simulink model "power_13NodeTestFeeder_4VSC_PV_DEG_symmtrc_loads_"  (R2024b)
settings: Solver=ode15s  StartTime=0.0  StopTime=5  FixedStep=1e-6  MaxStep=1e-4  RelTol=1e-6  AbsTol=1e-8  EnableMultiTasking=on
PreLoadFcn:
  | %power_13NodeTestFeeder_init;
values from neighbouring files (symbols this model uses):
  a = 1.3    [init_para_with_symmtrc_loads.m]
  Cdc = 278e-3    (= 0.278)    [init_para_with_symmtrc_loads.m]
  fg = 60    [a01_scan_VSC_13_feeder.m]    (also in init_para_with_symmtrc_loads.m)
  Gn = 1000    [init_para_with_symmtrc_loads.m]
  H = 8    [init_para_with_symmtrc_loads.m]
  Ipv_n = Isc_n*(Rp+Rs)/Rp    (= 8.21426513558)    [init_para_with_symmtrc_loads.m]
  Isc_n = 8.21    [init_para_with_symmtrc_loads.m]
  k = 1.3806503e-23    [init_para_with_symmtrc_loads.m]    (also in ypm_plot_compare_ana_meas.m = 2)
  Kdroop = Sn/(Rdroop*60)    (= 4166666.66667)    [init_para_with_symmtrc_loads.m]
  KI = 0.0032    [init_para_with_symmtrc_loads.m]
  Ki_C = Rc/tau_C    (= 0.768)    [init_para_with_symmtrc_loads.m]
  Ki_DC = omega_DC^2*Cdc    [init_para_with_symmtrc_loads.m]
  ki_dvpp = kp_dvpp/Ti_dvpp    [init_para_with_symmtrc_loads.m]
  Ki_P = 1/(Ki_pq*tau_P)    [init_para_with_symmtrc_loads.m]
  Ki_PLL = Kp_PLL/tau_PLL    [init_para_with_symmtrc_loads.m]
  Kp_C = Lc/tau_C    (= 0.020372)    [init_para_with_symmtrc_loads.m]
  Kp_DC = 2*xi_DC*omega_DC*Cdc    [init_para_with_symmtrc_loads.m]
  kp_dvpp = -(2*Kdcgain)^-1    [init_para_with_symmtrc_loads.m]
  Kp_P = tau_C/(Ki_pq*tau_P)    [init_para_with_symmtrc_loads.m]
  Kp_PLL = xi_PLL*2*omega_PLL/Vp    [init_para_with_symmtrc_loads.m]
  KV = -0.123    [init_para_with_symmtrc_loads.m]
  kv_Vp = [ 1.021 1.042 1.0174]    [init_para_with_symmtrc_loads.m]
  KVmp = Vmp_n/Voc_n    (= 0.799392097264)    [init_para_with_symmtrc_loads.m]
  Lc = 20.372e-6    (= 2.0372e-05)    [init_para_with_symmtrc_loads.m]
  Lg = Xg /(2*pi*fg)    [init_para_with_symmtrc_loads.m]
  Np = 345    [init_para_with_symmtrc_loads.m]
  Ns = 45    [init_para_with_symmtrc_loads.m]
  Ns_cell = 54    [init_para_with_symmtrc_loads.m]
  p_jump_time = 5    [init_para_with_symmtrc_loads.m]
  p_jump_value = 2*-1e6    (= -2000000)    [init_para_with_symmtrc_loads.m]
  phi_vec = phi_vec_deg/180*pi    [init_para_with_symmtrc_loads.m]
  ppv_nom = 4.9687e+05    (= 496870)    [init_para_with_symmtrc_loads.m]
  q = 1.6021764e-19    [init_para_with_symmtrc_loads.m]
  Rc = 0.768e-3    (= 0.000768)    [init_para_with_symmtrc_loads.m]
  Rg = (U_rms^2 / S_sc) / (sqrt(1 + XoverR^2))    [init_para_with_symmtrc_loads.m]
  Rp = 425.405    [init_para_with_symmtrc_loads.m]
  Rs = 0.221    [init_para_with_symmtrc_loads.m]
  S_base_all = 1    [init_para_with_symmtrc_loads.m]
  Sn = 15e6    (= 15000000)    [init_para_with_symmtrc_loads.m]
  tau_PLL = 2*xi_PLL/omega_PLL    [init_para_with_symmtrc_loads.m]
  Tn = 25    [init_para_with_symmtrc_loads.m]
  Ts = T_ctrl/n_ctrl    [a01_scan_VSC_13_feeder.m]    (also in init_para_with_symmtrc_loads.m = 5e-05)
  U_rms = 4160    [init_para_with_symmtrc_loads.m]
  Vdc = 1200    [init_para_with_symmtrc_loads.m]
  Voc_n = 32.9    [init_para_with_symmtrc_loads.m]
  Vp = sqrt(2)*480/sqrt(3)    [a01_scan_VSC_13_feeder.m]    (also in init_para_with_symmtrc_loads.m = Ug*sqrt(2)/sqrt(3))
undefined symbols (not defined in the file or in its folder): j, Newton, para_grid, para_PVgeno, Raphson
libraries: spsabctoAlphaBetaZeroLib x141, spsPower3phInstantaneousLib x70, spsSeriesRLCBranchLib x44, spsThreePhaseVIMeasurementLib x27, slpidlib x24, spsThreePhaseSeriesRLCLoadLib x15, spsControlledVoltageSourceLib x15, spsMeanLib x9, spsCurrentMeasurementLib x8, spsControlledCurrentSourceLib x8, cstblocks x8, spsGroundLib x5
(part 2 of 10)

== system power_13NodeTestFeeder_4VSC_PV_DEG_symmtrc_loads_/PV1 dynamic Load2 ==
  delta_p : Inport
  Bus Selector : BusSelector  OutputSignals=Active power P (W)
  Constant : Constant  Value=ppv_nom
  Gain : Gain  Gain=[-1 0]
  PVG_at_634 : spsThreePhaseVIMeasurementLib/Three-Phase V-I Measurement  VoltageMeasurement=phase-to-ground  SetLabelV=off  LabelV=Vabc_634_pv  Vpu=off  VpuLL=off  CurrentMeasurement=yes  SetLabelI=off  LabelI=Iabc_634_pv  Ipu=off  Pbase=100e6  Vbase=4160  OutputType=Complex  PhasorSimulation=off  PSBequivalent=0
  Scope3 : Scope
  Sum : Sum  Inputs=|++
  Three-Phase Dynamic Load : spsThreePhaseDynamicLoadLib/Three-Phase Dynamic Load  NominalVoltage=[ para_grid.n634YgPQ.V_LN_rms(1)*sqrt(3) 60 ]  ActiveReactivePowers=[ppv_nom 0]  PositiveSequence=[1 0]  ExternalControl=on  NpNq=[1.3 2]  TimeConstants="[0  0  0  0]"  MinimumVoltage=0.7  Tfilter=1e-4  LoadFlowParameters=[4,0,0,0,0]
  a : PMIOPort  Side=Right
  b : PMIOPort  Port=2  Side=Right
  c : PMIOPort  Port=3  Side=Right
  tag scope: Iabc_675_pv=global, Vabc_675_pv=global
  wires:
  PVG_at_634/1 -> [Vabc_675_pv]
  Bus Selector/1 -> Scope3/1  "<Active power P (W)>"
  PVG_at_634/2 -> [Iabc_675_pv]
  Three-Phase Dynamic Load/1 -> Bus Selector/1
  Constant/1 -> Sum/2
  Gain/1 -> Three-Phase Dynamic Load/1
  Sum/1 -> Gain/1
  delta_p/1 -> Sum/1
  connections:
  PVG_at_634/LConn3 -- Three-Phase Dynamic Load/LConn3
  b/RConn1 -- PVG_at_634/RConn2
  a/RConn1 -- PVG_at_634/RConn1
  PVG_at_634/LConn2 -- Three-Phase Dynamic Load/LConn2
  c/RConn1 -- PVG_at_634/RConn3
  PVG_at_634/LConn1 -- Three-Phase Dynamic Load/LConn1

== system power_13NodeTestFeeder_4VSC_PV_DEG_symmtrc_loads_/PV1 dynamic Load3 ==
  delta_p : Inport
  Bus Selector : BusSelector  OutputSignals=Active power P (W)
  Constant : Constant  Value=ppv_nom
  Gain : Gain  Gain=[-1 0]
  PVG_at_634 : spsThreePhaseVIMeasurementLib/Three-Phase V-I Measurement  VoltageMeasurement=phase-to-ground  SetLabelV=off  LabelV=Vabc_634_pv  Vpu=off  VpuLL=off  CurrentMeasurement=yes  SetLabelI=off  LabelI=Iabc_634_pv  Ipu=off  Pbase=100e6  Vbase=4160  OutputType=Complex  PhasorSimulation=off  PSBequivalent=0
  Scope3 : Scope
  Sum : Sum  Inputs=|++
  Three-Phase Dynamic Load : spsThreePhaseDynamicLoadLib/Three-Phase Dynamic Load  NominalVoltage=[ para_grid.n634YgPQ.V_LN_rms(1)*sqrt(3) 60 ]  ActiveReactivePowers=[ppv_nom 0]  PositiveSequence=[1 0]  ExternalControl=on  NpNq=[1.3 2]  TimeConstants="[0  0  0  0]"  MinimumVoltage=0.7  Tfilter=1e-4  LoadFlowParameters=[4,0,0,0,0]
  a : PMIOPort  Side=Right
  b : PMIOPort  Port=2  Side=Right
  c : PMIOPort  Port=3  Side=Right
  tag scope: Iabc_680_pv=global, Vabc_680_pv=global
  wires:
  PVG_at_634/1 -> [Vabc_680_pv]
  Bus Selector/1 -> Scope3/1  "<Active power P (W)>"
  PVG_at_634/2 -> [Iabc_680_pv]
  Three-Phase Dynamic Load/1 -> Bus Selector/1
  Constant/1 -> Sum/2
  Gain/1 -> Three-Phase Dynamic Load/1
  Sum/1 -> Gain/1
  delta_p/1 -> Sum/1
  connections:
  PVG_at_634/LConn3 -- Three-Phase Dynamic Load/LConn3
  b/RConn1 -- PVG_at_634/RConn2
  a/RConn1 -- PVG_at_634/RConn1
  PVG_at_634/LConn2 -- Three-Phase Dynamic Load/LConn2
  c/RConn1 -- PVG_at_634/RConn3
  PVG_at_634/LConn1 -- Three-Phase Dynamic Load/LConn1

== system power_13NodeTestFeeder_4VSC_PV_DEG_symmtrc_loads_/PV2 dynamic Load ==
  delta_p : Inport
  Bus Selector : BusSelector  OutputSignals=Active power P (W)
  Constant : Constant  Value=ppv_nom
  Gain : Gain  Gain=[-1 0]
  PVG_at_634 : spsThreePhaseVIMeasurementLib/Three-Phase V-I Measurement  VoltageMeasurement=phase-to-ground  SetLabelV=off  LabelV=Vabc_634_pv  Vpu=off  VpuLL=off  CurrentMeasurement=yes  SetLabelI=off  LabelI=Iabc_634_pv  Ipu=off  Pbase=100e6  Vbase=4160  OutputType=Complex  PhasorSimulation=off  PSBequivalent=0
  Scope3 : Scope
  Sum : Sum  Inputs=|++
  Three-Phase Dynamic Load : spsThreePhaseDynamicLoadLib/Three-Phase Dynamic Load  NominalVoltage=[ para_grid.n634YgPQ.V_LN_rms(1)*sqrt(3) 60 ]  ActiveReactivePowers=[ppv_nom 0]  PositiveSequence=[1 0]  ExternalControl=on  NpNq=[1.3 2]  TimeConstants="[0  0  0  0]"  MinimumVoltage=0.7  Tfilter=1e-4  LoadFlowParameters=[4,0,0,0,0]
  a : PMIOPort  Side=Right
  b : PMIOPort  Port=2  Side=Right
  c : PMIOPort  Port=3  Side=Right
  tag scope: Iabc_672_pv=global, Vabc_672_pv=global
  wires:
  PVG_at_634/1 -> [Vabc_672_pv]
  Bus Selector/1 -> Scope3/1  "<Active power P (W)>"
  PVG_at_634/2 -> [Iabc_672_pv]
  Three-Phase Dynamic Load/1 -> Bus Selector/1
  Constant/1 -> Sum/2
  Gain/1 -> Three-Phase Dynamic Load/1
  delta_p/1 -> Sum/1
  Sum/1 -> Gain/1
  connections:
  PVG_at_634/LConn3 -- Three-Phase Dynamic Load/LConn3
  b/RConn1 -- PVG_at_634/RConn2
  a/RConn1 -- PVG_at_634/RConn1
  PVG_at_634/LConn2 -- Three-Phase Dynamic Load/LConn2
  c/RConn1 -- PVG_at_634/RConn3
  PVG_at_634/LConn1 -- Three-Phase Dynamic Load/LConn1

== system power_13NodeTestFeeder_4VSC_PV_DEG_symmtrc_loads_/PV_Geno_GFL_VSC_at_634 ==
  note: 5.23e5
  "PV-Geno with VSC_GFL_at_634     " : Subsystem
      settings: PortSchema="{\"entries\":[{\"content\":{\"sides\":[{\"content\":{\"connectorIds\":[\"LConn1\",\"LConn2\",\"LConn3\"]},\"type\":\"ConnectorPlacement.EquallySpacedRectSide\",\"uuid\":\"92a05cf9-a19b-475d-bffb-9406018f82f4\"},{\"content\":{\"connectorIds\":[\"In1\",\"In2\",\"In3\"],\"side\":\"RIGHT\"},\"type\":\"ConnectorPlacement.EquallySpacedRectSide\",\"uuid\":\"83076eb6-0a86-49d7-8932-035501cdc6f6\"},{\"content\":{\"side\":\"TOP\"},\"type\":\"ConnectorPlacement.EquallySpacedRectSide\",\"uuid\":\"ba2310df-ee07-4a5c-88ff-ef0f81658322\"}]},\"type\":\"ConnectorPlacement.EquallySpacedConnector\",\"uuid\":\"9e64c472-0dae-4bb4-8eb3-3329c328d412\"}],\"packageUris\":[\"http://schema.mathworks.com/mf0/Connector/R2020b\"],\"version\":\"1.0\"}"
  PVG_at_634 : spsThreePhaseVIMeasurementLib/Three-Phase V-I Measurement  VoltageMeasurement=phase-to-ground  SetLabelV=off  LabelV=Vabc_634_pv  Vpu=off  VpuLL=off  CurrentMeasurement=yes  SetLabelI=off  LabelI=Iabc_634_pv  Ipu=off  Pbase=100e6  Vbase=4160  OutputType=Complex  PhasorSimulation=off  PSBequivalent=0
  S Signalgenerator_at_1 : Subsystem
  a : PMIOPort  Side=Right
  b : PMIOPort  Port=2  Side=Right
  c : PMIOPort  Port=3  Side=Right
  tag scope: Iabc_634_pv=global, Vabc_634_pv=global
  wires:
  S Signalgenerator_at_1/1(S) -> "PV-Geno with VSC_GFL_at_634     "/3(S)
  PVG_at_634/2 -> [Iabc_634_pv], "PV-Geno with VSC_GFL_at_634     "/2(I_abc)
  PVG_at_634/1 -> [Vabc_634_pv], "PV-Geno with VSC_GFL_at_634     "/1(V_abc)
  connections:
  PVG_at_634/RConn2 -- b/RConn1
  "PV-Geno with VSC_GFL_at_634     "/LConn3 -- PVG_at_634/LConn3
  "PV-Geno with VSC_GFL_at_634     "/LConn1 -- PVG_at_634/LConn1
  "PV-Geno with VSC_GFL_at_634     "/LConn2 -- PVG_at_634/LConn2
  PVG_at_634/RConn1 -- a/RConn1
  PVG_at_634/RConn3 -- c/RConn1

== system power_13NodeTestFeeder_4VSC_PV_DEG_symmtrc_loads_/PV_Geno_GFL_VSC_at_672 ==
  PV-Geno with VSC_GFL_at_672 : Subsystem
      settings: PortSchema="{\"entries\":[{\"content\":{\"sides\":[{\"content\":{\"connectorIds\":[\"LConn1\",\"LConn2\",\"LConn3\"]},\"type\":\"ConnectorPlacement.EquallySpacedRectSide\",\"uuid\":\"92a05cf9-a19b-475d-bffb-9406018f82f4\"},{\"content\":{\"connectorIds\":[\"In1\",\"In2\",\"In3\"],\"side\":\"RIGHT\"},\"type\":\"ConnectorPlacement.EquallySpacedRectSide\",\"uuid\":\"83076eb6-0a86-49d7-8932-035501cdc6f6\"},{\"content\":{\"side\":\"TOP\"},\"type\":\"ConnectorPlacement.EquallySpacedRectSide\",\"uuid\":\"ba2310df-ee07-4a5c-88ff-ef0f81658322\"}]},\"type\":\"ConnectorPlacement.EquallySpacedConnector\",\"uuid\":\"9e64c472-0dae-4bb4-8eb3-3329c328d412\"}],\"packageUris\":[\"http://schema.mathworks.com/mf0/Connector/R2020b\"],\"version\":\"1.0\"}"
  S Signalgenerator_at_672 : Subsystem
  VSC_GFL_at_672 : spsThreePhaseVIMeasurementLib/Three-Phase V-I Measurement  VoltageMeasurement=phase-to-ground  SetLabelV=off  LabelV=Vabc_634  Vpu=off  VpuLL=off  CurrentMeasurement=yes  SetLabelI=off  LabelI=Iabc_634  Ipu=off  Pbase=100e6  Vbase=4160  OutputType=Complex  PhasorSimulation=off  PSBequivalent=0
  a : PMIOPort  Side=Right
  b : PMIOPort  Port=2  Side=Right
  c : PMIOPort  Port=3  Side=Right
  tag scope: Iabc_672_pv=global, Vabc_672_pv=global
  wires:
  VSC_GFL_at_672/2 -> [Iabc_672_pv], PV-Geno with VSC_GFL_at_672/2(I_abc)
  VSC_GFL_at_672/1 -> [Vabc_672_pv], PV-Geno with VSC_GFL_at_672/1(V_abc)
  S Signalgenerator_at_672/1(S) -> PV-Geno with VSC_GFL_at_672/3(S)
  connections:
  PV-Geno with VSC_GFL_at_672/LConn1 -- VSC_GFL_at_672/LConn1
  PV-Geno with VSC_GFL_at_672/LConn3 -- VSC_GFL_at_672/LConn3
  PV-Geno with VSC_GFL_at_672/LConn2 -- VSC_GFL_at_672/LConn2
  a/RConn1 -- VSC_GFL_at_672/RConn1
  c/RConn1 -- VSC_GFL_at_672/RConn3
  b/RConn1 -- VSC_GFL_at_672/RConn2

== system power_13NodeTestFeeder_4VSC_PV_DEG_symmtrc_loads_/PV_Geno_GFL_VSC_at_675 ==
  PV-Geno with VSC_GFL_at_675 : Subsystem
      settings: PortSchema="{\"entries\":[{\"content\":{\"sides\":[{\"content\":{\"connectorIds\":[\"LConn1\",\"LConn2\",\"LConn3\"]},\"type\":\"ConnectorPlacement.EquallySpacedRectSide\",\"uuid\":\"92a05cf9-a19b-475d-bffb-9406018f82f4\"},{\"content\":{\"connectorIds\":[\"In1\",\"In2\",\"In3\"],\"side\":\"RIGHT\"},\"type\":\"ConnectorPlacement.EquallySpacedRectSide\",\"uuid\":\"83076eb6-0a86-49d7-8932-035501cdc6f6\"},{\"content\":{\"side\":\"TOP\"},\"type\":\"ConnectorPlacement.EquallySpacedRectSide\",\"uuid\":\"ba2310df-ee07-4a5c-88ff-ef0f81658322\"}]},\"type\":\"ConnectorPlacement.EquallySpacedConnector\",\"uuid\":\"9e64c472-0dae-4bb4-8eb3-3329c328d412\"}],\"packageUris\":[\"http://schema.mathworks.com/mf0/Connector/R2020b\"],\"version\":\"1.0\"}"
  PVG_at_675 : spsThreePhaseVIMeasurementLib/Three-Phase V-I Measurement  VoltageMeasurement=phase-to-ground  SetLabelV=off  LabelV=Vabc_634  Vpu=off  VpuLL=off  CurrentMeasurement=yes  SetLabelI=off  LabelI=Iabc_634  Ipu=off  Pbase=100e6  Vbase=4160  OutputType=Complex  PhasorSimulation=off  PSBequivalent=0
  S Signalgenerator_at_675 : Subsystem
  v_a : PMIOPort  Side=Right
  v_b : PMIOPort  Port=2  Side=Right
  v_c : PMIOPort  Port=3  Side=Right
  tag scope: Iabc_675_pv=global, Vabc_675_pv=global
  wires:
  PVG_at_675/2 -> [Iabc_675_pv], PV-Geno with VSC_GFL_at_675/2(I_abc)
  PVG_at_675/1 -> [Vabc_675_pv], PV-Geno with VSC_GFL_at_675/1(V_abc)
  S Signalgenerator_at_675/1(S) -> PV-Geno with VSC_GFL_at_675/3(S)
  connections:
  PV-Geno with VSC_GFL_at_675/LConn3 -- PVG_at_675/LConn3
  PVG_at_675/RConn2 -- v_b/RConn1
  PVG_at_675/RConn1 -- v_a/RConn1
  PV-Geno with VSC_GFL_at_675/LConn1 -- PVG_at_675/LConn1
  PV-Geno with VSC_GFL_at_675/LConn2 -- PVG_at_675/LConn2
  PVG_at_675/RConn3 -- v_c/RConn1

== system power_13NodeTestFeeder_4VSC_PV_DEG_symmtrc_loads_/PV_Geno_GFL_VSC_at_680 ==
  PV-Geno with VSC_GFL_at_680 : Subsystem
      settings: PortSchema="{\"entries\":[{\"content\":{\"sides\":[{\"content\":{\"connectorIds\":[\"LConn1\",\"LConn2\",\"LConn3\"]},\"type\":\"ConnectorPlacement.EquallySpacedRectSide\",\"uuid\":\"92a05cf9-a19b-475d-bffb-9406018f82f4\"},{\"content\":{\"connectorIds\":[\"In1\",\"In2\",\"In3\"],\"side\":\"RIGHT\"},\"type\":\"ConnectorPlacement.EquallySpacedRectSide\",\"uuid\":\"83076eb6-0a86-49d7-8932-035501cdc6f6\"},{\"content\":{\"side\":\"TOP\"},\"type\":\"ConnectorPlacement.EquallySpacedRectSide\",\"uuid\":\"ba2310df-ee07-4a5c-88ff-ef0f81658322\"}]},\"type\":\"ConnectorPlacement.EquallySpacedConnector\",\"uuid\":\"9e64c472-0dae-4bb4-8eb3-3329c328d412\"}],\"packageUris\":[\"http://schema.mathworks.com/mf0/Connector/R2020b\"],\"version\":\"1.0\"}"
  PVG_at_680 : spsThreePhaseVIMeasurementLib/Three-Phase V-I Measurement  VoltageMeasurement=phase-to-ground  SetLabelV=off  LabelV=Vabc_634  Vpu=off  VpuLL=off  CurrentMeasurement=yes  SetLabelI=off  LabelI=Iabc_634  Ipu=off  Pbase=100e6  Vbase=4160  OutputType=Complex  PhasorSimulation=off  PSBequivalent=0
  S Signalgenerator_at_680 : Subsystem
  a : PMIOPort  Side=Right
  b : PMIOPort  Port=2  Side=Right
  c : PMIOPort  Port=3  Side=Right
  tag scope: Iabc_680_pv=global, Vabc_680_pv=global
  wires:
  PVG_at_680/2 -> [Iabc_680_pv], PV-Geno with VSC_GFL_at_680/2(I_abc)
  PVG_at_680/1 -> [Vabc_680_pv], PV-Geno with VSC_GFL_at_680/1(V_abc)
  S Signalgenerator_at_680/1(S) -> PV-Geno with VSC_GFL_at_680/3(S)
  connections:
  PVG_at_680/RConn3 -- c/RConn1
  PV-Geno with VSC_GFL_at_680/LConn2 -- PVG_at_680/LConn2
  PVG_at_680/LConn1 -- PV-Geno with VSC_GFL_at_680/LConn1
  PVG_at_680/RConn2 -- b/RConn1
  PV-Geno with VSC_GFL_at_680/LConn3 -- PVG_at_680/LConn3
  PVG_at_680/RConn1 -- a/RConn1

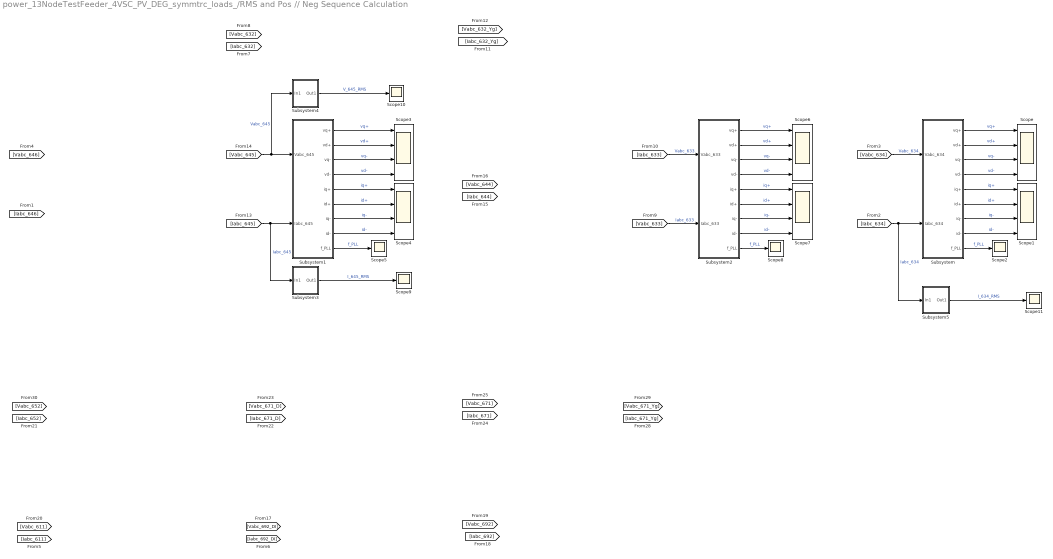
== system power_13NodeTestFeeder_4VSC_PV_DEG_symmtrc_loads_/RMS and Pos // Neg Sequence Calculation  ==
  Scope{,1,3..4,6..7} (6 alike) : Scope  NumInputPorts=4
  Scope{2,5,8..11} (6 alike) : Scope
  Subsystem : Subsystem
  Subsystem1 : Subsystem
  Subsystem2 : Subsystem
  Subsystem3 : Subsystem  mask{fg=fg, Vrms0=0}
      mask prompts: fg "Frequency"; Vrms0 "Initial value"
      mask Display: disp('RMS')
  Subsystem4 : Subsystem  mask{fg=fg, Vrms0=0}
      mask prompts: fg "Frequency"; Vrms0 "Initial value"
      mask Display: disp('RMS')
  Subsystem5 : Subsystem  mask{fg=fg, Vrms0=0}
      mask prompts: fg "Frequency"; Vrms0 "Initial value"
      mask Display: disp('RMS')
  wires:
  [Vabc_634] -> Subsystem/1(Vabc_634)  "Vabc_634"
  [Iabc_634] -> Subsystem5/1(In1), Subsystem/2(Iabc_634)  "Iabc_634"
  Subsystem/1(vq+) -> Scope/1  "vq+"
  Subsystem/2(vd+) -> Scope/2  "vd+"
  Subsystem/3(vq-) -> Scope/3  "vq-"
  Subsystem/4(vd-) -> Scope/4  "vd-"
  Subsystem/9(f_PLL) -> Scope2/1  "f_PLL"
  Subsystem/5(iq+) -> Scope1/1  "iq+"
  Subsystem/6(id+) -> Scope1/2  "id+"
  Subsystem/7(iq-) -> Scope1/3  "iq-"
  Subsystem/8(id-) -> Scope1/4  "id-"
  Subsystem1/6(id+) -> Scope4/2  "id+"
  Subsystem1/8(id-) -> Scope4/4  "id-"
  Subsystem1/7(iq-) -> Scope4/3  "iq-"
  [Vabc_645] -> Subsystem1/1(Vabc_645), Subsystem4/1(In1)  "Vabc_645"
  Subsystem1/1(vq+) -> Scope3/1  "vq+"
  Subsystem1/5(iq+) -> Scope4/1  "iq+"
  [Iabc_645] -> Subsystem3/1(In1), Subsystem1/2(Iabc_645)  "Iabc_645"
  Subsystem1/2(vd+) -> Scope3/2  "vd+"
  Subsystem1/9(f_PLL) -> Scope5/1  "f_PLL"
  Subsystem1/3(vq-) -> Scope3/3  "vq-"
  Subsystem1/4(vd-) -> Scope3/4  "vd-"
  Subsystem2/6(id+) -> Scope7/2  "id+"
  Subsystem2/8(id-) -> Scope7/4  "id-"
  Subsystem2/7(iq-) -> Scope7/3  "iq-"
  [Iabc_633] -> Subsystem2/1(Vabc_633)  "Vabc_633"
  Subsystem2/1(vq+) -> Scope6/1  "vq+"
  Subsystem2/5(iq+) -> Scope7/1  "iq+"
  [Vabc_633] -> Subsystem2/2(Iabc_633)  "Iabc_633"
  Subsystem2/2(vd+) -> Scope6/2  "vd+"
  Subsystem2/9(f_PLL) -> Scope8/1  "f_PLL"
  Subsystem2/3(vq-) -> Scope6/3  "vq-"
  Subsystem2/4(vd-) -> Scope6/4  "vd-"
  Subsystem3/1(Out1) -> Scope9/1  "I_645_RMS"
  Subsystem4/1(Out1) -> Scope10/1  "V_645_RMS"
  Subsystem5/1(Out1) -> Scope11/1  "I_634_RMS"

== system power_13NodeTestFeeder_4VSC_PV_DEG_symmtrc_loads_/Subsystem ==
  dPreq : Inport
  Constant : Constant
  Constant1 : Constant  Value=0
  Gain : Gain  Gain=-1
  Switch1 : Switch  Criteria=u2 > Threshold  SaturateOnIntegerOverflow=off  InputSameDT=off
  dPchange : Outport
  wires:
  Constant/1 -> Switch1/1
  Switch1/1 -> dPchange/1
  dPreq/1 -> Gain/1
  Constant1/1 -> Switch1/3
  Gain/1 -> Switch1/2

== system power_13NodeTestFeeder_4VSC_PV_DEG_symmtrc_loads_/Tagg5 ==
  df : Inport
  LTI System1 : cstblocks/LTI System  Commented=on  sys=T_pf_agg  IC=[]  PadeOrder=0
  LTI System8 : cstblocks/LTI System  sys=m1  IC=[]  PadeOrder=0
  Multiply : Gain  Gain=ppv_nom
  PID Controller : slpidlib/PID Controller  Controller=PI  Form=Parallel  TimeDomain=Continuous-time  UseExternalTs=off  SampleTime=-1  IntegratorMethod=Forward Euler  FilterMethod=Forward Euler  ControllerParametersSource=internal  P=kp_dvpp  I=ki_dvpp  UseKiTs=off  D=0  UseExternalDerivativeSource=off  N=100  UseFilter=on  TunerSelectOption=Transfer Function Based (PID Tuner App)  InitialConditionSource=internal  InitialConditionForIntegrator=0  InitialConditionForFilter=0  DifferentiatorICPrevScaledInput=0  ExternalReset=either  TrackingMode=off  Kt=1  LimitOutput=off  SatLimitsSource=internal  UpperSaturationLimit=inf  LowerSaturationLimit=-inf  LinearizeAsGain=on  AntiWindupMode=none  Kb=1  LimitIntegrator=off  UpperIntegratorSaturationLimit=inf  LowerIntegratorSaturationLimit=-inf  POutMin=[]  POutMax=[]  IOutMin=[]  IOutMax=[]  DOutMin=[]  DOutMax=[]  NOutMin=[]  NOutMax=[]  SumOutMin=[]  SumOutMax=[]  SaturationOutMin=[]  SaturationOutMax=[]  PParamMin=[]  PParamMax=[]  IParamMin=[]  IParamMax=[]  DParamMin=[]  DParamMax=[]  NParamMin=[]  NParamMax=[]  KbParamMin=[]  KbParamMax=[]  KtParamMin=[]  KtParamMax=[]  KbOutMin=[]  KbOutMax=[]  KtOutMin=[]  KtOutMax=[]  IntegratorOutMin=[]  IntegratorOutMax=[]  FilterOutMin=[]  FilterOutMax=[]  SumI1OutMin=[]  SumI1OutMax=[]  SumI2OutMin=[]  SumI2OutMax=[]  SumI3OutMin=[]  SumI3OutMax=[]  SumI4OutMin=[]  SumI4OutMax=[]  SumDOutMin=[]  SumDOutMax=[]  DifferentiatorOutMin=[]  DifferentiatorOutMax=[]  FilterDiffOutCoefMin=[]  FilterDiffOutCoefMax=[]  ReciprocalOutMin=[]  ReciprocalOutMax=[]  SumDenOutMin=[]  SumDenOutMax=[]  SumNumOutMin=[]  SumNumOutMax=[]  DivideOutMin=[]  DivideOutMax=[]  UdiffTsProdOutMin=[]  UdiffTsProdOutMax=[]  NTsProdOutMin=[]  NTsProdOutMax=[]  UintegralTsProdOutMin=[]  UintegralTsProdOutMax=[]  UngainTsProdOutMin=[]  UngainTsProdOutMax=[]  ClampingZeroOutDataTypeStr=Inherit: Inherit via back propagation  ClampingZeroOutMin=[]  ClampingZeroOutMax=[]  FilterDenConstantOutDataTypeStr=Inherit: Inherit via back propagation  FilterDenConstantOutMin=[]  FilterDenConstantOutMax=[]  PCopyOutDataTypeStr=Inherit: Inherit via back propagation  PCopyOutMin=[]  PCopyOutMax=[]  NCopyOutDataTypeStr=Inherit: Inherit via back propagation  NCopyOutMin=[]  NCopyOutMax=[]  IntegratorContinuousStateAttributes=''  IntegratorStateMustResolveToSignalObject=off  IntegratorRTWStateStorageClass=Auto  FilterContinuousStateAttributes=''  FilterStateMustResolveToSignalObject=off  FilterRTWStateStorageClass=Auto  ParallelPVariant=InternalParameters  IdealPVariant=Disabled  IVariant=InternalParameters  DVariant=Disabled  IntegratorVariant=Continuous  SatVariant=Disabled  AWVariant=Passthrough  PCopyVariant=Disabled  TRVariant=Disabled  FdbkBlocksVariant=Forward  IdealPFdbkVariant=Disabled  SatFdbkVariant=Disabled  DerivativeFilterVariant=Disabled  NVariant=Disabled  NCopyVariant=Disabled_SignalSpec  FilterICVariant=Disabled  IntegratorICVariant=InternalICs  ExternalResetVariant=ExternalReset  TRSumVariant=Passthrough  SumFdbkVariant=Disabled  SumVariant=Sum_PI  TsampFilterVariant=InternalTs  TsampNgainVariant=Passthrough  TsampIntegralVariant=Disabled_SignalSpec  ExternalSaturationOutDataTypeStr=Inherit: Same as second input  DerivativeSourceVariant=Disabled  PreIntVariant=InternalPreInt
  dP : Outport
  tag scope: m1=global
  wires:
  Multiply/1 -> dP/1
  df/1 -> LTI System8/1
  LTI System8/1 -> [m1], PID Controller/1
  PID Controller/1 -> Multiply/1
  [resetI] -> PID Controller/2

== system power_13NodeTestFeeder_4VSC_PV_DEG_symmtrc_loads_/Tagg6 ==
  df : Inport
  LTI System1 : cstblocks/LTI System  Commented=on  sys=T_pf_agg  IC=[]  PadeOrder=0
  LTI System8 : cstblocks/LTI System  sys=m3  IC=[]  PadeOrder=0
  Multiply : Gain  Gain=ppv_nom
  PID Controller : slpidlib/PID Controller  Controller=PI  Form=Parallel  TimeDomain=Continuous-time  UseExternalTs=off  SampleTime=-1  IntegratorMethod=Forward Euler  FilterMethod=Forward Euler  ControllerParametersSource=internal  P=kp_dvpp  I=ki_dvpp  UseKiTs=off  D=0  UseExternalDerivativeSource=off  N=100  UseFilter=on  TunerSelectOption=Transfer Function Based (PID Tuner App)  InitialConditionSource=internal  InitialConditionForIntegrator=0  InitialConditionForFilter=0  DifferentiatorICPrevScaledInput=0  ExternalReset=either  TrackingMode=off  Kt=1  LimitOutput=off  SatLimitsSource=internal  UpperSaturationLimit=inf  LowerSaturationLimit=-inf  LinearizeAsGain=on  AntiWindupMode=none  Kb=1  LimitIntegrator=off  UpperIntegratorSaturationLimit=inf  LowerIntegratorSaturationLimit=-inf  POutMin=[]  POutMax=[]  IOutMin=[]  IOutMax=[]  DOutMin=[]  DOutMax=[]  NOutMin=[]  NOutMax=[]  SumOutMin=[]  SumOutMax=[]  SaturationOutMin=[]  SaturationOutMax=[]  PParamMin=[]  PParamMax=[]  IParamMin=[]  IParamMax=[]  DParamMin=[]  DParamMax=[]  NParamMin=[]  NParamMax=[]  KbParamMin=[]  KbParamMax=[]  KtParamMin=[]  KtParamMax=[]  KbOutMin=[]  KbOutMax=[]  KtOutMin=[]  KtOutMax=[]  IntegratorOutMin=[]  IntegratorOutMax=[]  FilterOutMin=[]  FilterOutMax=[]  SumI1OutMin=[]  SumI1OutMax=[]  SumI2OutMin=[]  SumI2OutMax=[]  SumI3OutMin=[]  SumI3OutMax=[]  SumI4OutMin=[]  SumI4OutMax=[]  SumDOutMin=[]  SumDOutMax=[]  DifferentiatorOutMin=[]  DifferentiatorOutMax=[]  FilterDiffOutCoefMin=[]  FilterDiffOutCoefMax=[]  ReciprocalOutMin=[]  ReciprocalOutMax=[]  SumDenOutMin=[]  SumDenOutMax=[]  SumNumOutMin=[]  SumNumOutMax=[]  DivideOutMin=[]  DivideOutMax=[]  UdiffTsProdOutMin=[]  UdiffTsProdOutMax=[]  NTsProdOutMin=[]  NTsProdOutMax=[]  UintegralTsProdOutMin=[]  UintegralTsProdOutMax=[]  UngainTsProdOutMin=[]  UngainTsProdOutMax=[]  ClampingZeroOutDataTypeStr=Inherit: Inherit via back propagation  ClampingZeroOutMin=[]  ClampingZeroOutMax=[]  FilterDenConstantOutDataTypeStr=Inherit: Inherit via back propagation  FilterDenConstantOutMin=[]  FilterDenConstantOutMax=[]  PCopyOutDataTypeStr=Inherit: Inherit via back propagation  PCopyOutMin=[]  PCopyOutMax=[]  NCopyOutDataTypeStr=Inherit: Inherit via back propagation  NCopyOutMin=[]  NCopyOutMax=[]  IntegratorContinuousStateAttributes=''  IntegratorStateMustResolveToSignalObject=off  IntegratorRTWStateStorageClass=Auto  FilterContinuousStateAttributes=''  FilterStateMustResolveToSignalObject=off  FilterRTWStateStorageClass=Auto  ParallelPVariant=InternalParameters  IdealPVariant=Disabled  IVariant=InternalParameters  DVariant=Disabled  IntegratorVariant=Continuous  SatVariant=Disabled  AWVariant=Passthrough  PCopyVariant=Disabled  TRVariant=Disabled  FdbkBlocksVariant=Forward  IdealPFdbkVariant=Disabled  SatFdbkVariant=Disabled  DerivativeFilterVariant=Disabled  NVariant=Disabled  NCopyVariant=Disabled_SignalSpec  FilterICVariant=Disabled  IntegratorICVariant=InternalICs  ExternalResetVariant=ExternalReset  TRSumVariant=Passthrough  SumFdbkVariant=Disabled  SumVariant=Sum_PI  TsampFilterVariant=InternalTs  TsampNgainVariant=Passthrough  TsampIntegralVariant=Disabled_SignalSpec  ExternalSaturationOutDataTypeStr=Inherit: Same as second input  DerivativeSourceVariant=Disabled  PreIntVariant=InternalPreInt
  dP : Outport
  tag scope: m3=global
  wires:
  Multiply/1 -> dP/1
  df/1 -> LTI System8/1
  PID Controller/1 -> Multiply/1
  [resetI] -> PID Controller/2
  LTI System8/1 -> [m3], PID Controller/1

== system power_13NodeTestFeeder_4VSC_PV_DEG_symmtrc_loads_/Tagg7 ==
  df : Inport
  LTI System1 : cstblocks/LTI System  Commented=on  sys=T_pf_agg  IC=[]  PadeOrder=0
  LTI System8 : cstblocks/LTI System  sys=m2  IC=[]  PadeOrder=0
  Multiply : Gain  Gain=ppv_nom
  PID Controller : slpidlib/PID Controller  Controller=PI  Form=Parallel  TimeDomain=Continuous-time  UseExternalTs=off  SampleTime=-1  IntegratorMethod=Forward Euler  FilterMethod=Forward Euler  ControllerParametersSource=internal  P=kp_dvpp  I=ki_dvpp  UseKiTs=off  D=0  UseExternalDerivativeSource=off  N=100  UseFilter=on  TunerSelectOption=Transfer Function Based (PID Tuner App)  InitialConditionSource=internal  InitialConditionForIntegrator=0  InitialConditionForFilter=0  DifferentiatorICPrevScaledInput=0  ExternalReset=either  TrackingMode=off  Kt=1  LimitOutput=off  SatLimitsSource=internal  UpperSaturationLimit=inf  LowerSaturationLimit=-inf  LinearizeAsGain=on  AntiWindupMode=none  Kb=1  LimitIntegrator=off  UpperIntegratorSaturationLimit=inf  LowerIntegratorSaturationLimit=-inf  POutMin=[]  POutMax=[]  IOutMin=[]  IOutMax=[]  DOutMin=[]  DOutMax=[]  NOutMin=[]  NOutMax=[]  SumOutMin=[]  SumOutMax=[]  SaturationOutMin=[]  SaturationOutMax=[]  PParamMin=[]  PParamMax=[]  IParamMin=[]  IParamMax=[]  DParamMin=[]  DParamMax=[]  NParamMin=[]  NParamMax=[]  KbParamMin=[]  KbParamMax=[]  KtParamMin=[]  KtParamMax=[]  KbOutMin=[]  KbOutMax=[]  KtOutMin=[]  KtOutMax=[]  IntegratorOutMin=[]  IntegratorOutMax=[]  FilterOutMin=[]  FilterOutMax=[]  SumI1OutMin=[]  SumI1OutMax=[]  SumI2OutMin=[]  SumI2OutMax=[]  SumI3OutMin=[]  SumI3OutMax=[]  SumI4OutMin=[]  SumI4OutMax=[]  SumDOutMin=[]  SumDOutMax=[]  DifferentiatorOutMin=[]  DifferentiatorOutMax=[]  FilterDiffOutCoefMin=[]  FilterDiffOutCoefMax=[]  ReciprocalOutMin=[]  ReciprocalOutMax=[]  SumDenOutMin=[]  SumDenOutMax=[]  SumNumOutMin=[]  SumNumOutMax=[]  DivideOutMin=[]  DivideOutMax=[]  UdiffTsProdOutMin=[]  UdiffTsProdOutMax=[]  NTsProdOutMin=[]  NTsProdOutMax=[]  UintegralTsProdOutMin=[]  UintegralTsProdOutMax=[]  UngainTsProdOutMin=[]  UngainTsProdOutMax=[]  ClampingZeroOutDataTypeStr=Inherit: Inherit via back propagation  ClampingZeroOutMin=[]  ClampingZeroOutMax=[]  FilterDenConstantOutDataTypeStr=Inherit: Inherit via back propagation  FilterDenConstantOutMin=[]  FilterDenConstantOutMax=[]  PCopyOutDataTypeStr=Inherit: Inherit via back propagation  PCopyOutMin=[]  PCopyOutMax=[]  NCopyOutDataTypeStr=Inherit: Inherit via back propagation  NCopyOutMin=[]  NCopyOutMax=[]  IntegratorContinuousStateAttributes=''  IntegratorStateMustResolveToSignalObject=off  IntegratorRTWStateStorageClass=Auto  FilterContinuousStateAttributes=''  FilterStateMustResolveToSignalObject=off  FilterRTWStateStorageClass=Auto  ParallelPVariant=InternalParameters  IdealPVariant=Disabled  IVariant=InternalParameters  DVariant=Disabled  IntegratorVariant=Continuous  SatVariant=Disabled  AWVariant=Passthrough  PCopyVariant=Disabled  TRVariant=Disabled  FdbkBlocksVariant=Forward  IdealPFdbkVariant=Disabled  SatFdbkVariant=Disabled  DerivativeFilterVariant=Disabled  NVariant=Disabled  NCopyVariant=Disabled_SignalSpec  FilterICVariant=Disabled  IntegratorICVariant=InternalICs  ExternalResetVariant=ExternalReset  TRSumVariant=Passthrough  SumFdbkVariant=Disabled  SumVariant=Sum_PI  TsampFilterVariant=InternalTs  TsampNgainVariant=Passthrough  TsampIntegralVariant=Disabled_SignalSpec  ExternalSaturationOutDataTypeStr=Inherit: Same as second input  DerivativeSourceVariant=Disabled  PreIntVariant=InternalPreInt
  dP : Outport
  tag scope: m2=global
  wires:
  Multiply/1 -> dP/1
  df/1 -> LTI System8/1
  PID Controller/1 -> Multiply/1
  [resetI] -> PID Controller/2
  LTI System8/1 -> [m2], PID Controller/1

== system power_13NodeTestFeeder_4VSC_PV_DEG_symmtrc_loads_/Tagg8 ==
  df : Inport
  LTI System1 : cstblocks/LTI System  Commented=on  sys=T_pf_agg  IC=[]  PadeOrder=0
  LTI System8 : cstblocks/LTI System  sys=m4  IC=[]  PadeOrder=0
  Multiply : Gain  Gain=ppv_nom
  PID Controller : slpidlib/PID Controller  Controller=PI  Form=Parallel  TimeDomain=Continuous-time  UseExternalTs=off  SampleTime=-1  IntegratorMethod=Forward Euler  FilterMethod=Forward Euler  ControllerParametersSource=internal  P=kp_dvpp  I=ki_dvpp  UseKiTs=off  D=0  UseExternalDerivativeSource=off  N=100  UseFilter=on  TunerSelectOption=Transfer Function Based (PID Tuner App)  InitialConditionSource=internal  InitialConditionForIntegrator=0  InitialConditionForFilter=0  DifferentiatorICPrevScaledInput=0  ExternalReset=either  TrackingMode=off  Kt=1  LimitOutput=off  SatLimitsSource=internal  UpperSaturationLimit=inf  LowerSaturationLimit=-inf  LinearizeAsGain=on  AntiWindupMode=none  Kb=1  LimitIntegrator=off  UpperIntegratorSaturationLimit=inf  LowerIntegratorSaturationLimit=-inf  POutMin=[]  POutMax=[]  IOutMin=[]  IOutMax=[]  DOutMin=[]  DOutMax=[]  NOutMin=[]  NOutMax=[]  SumOutMin=[]  SumOutMax=[]  SaturationOutMin=[]  SaturationOutMax=[]  PParamMin=[]  PParamMax=[]  IParamMin=[]  IParamMax=[]  DParamMin=[]  DParamMax=[]  NParamMin=[]  NParamMax=[]  KbParamMin=[]  KbParamMax=[]  KtParamMin=[]  KtParamMax=[]  KbOutMin=[]  KbOutMax=[]  KtOutMin=[]  KtOutMax=[]  IntegratorOutMin=[]  IntegratorOutMax=[]  FilterOutMin=[]  FilterOutMax=[]  SumI1OutMin=[]  SumI1OutMax=[]  SumI2OutMin=[]  SumI2OutMax=[]  SumI3OutMin=[]  SumI3OutMax=[]  SumI4OutMin=[]  SumI4OutMax=[]  SumDOutMin=[]  SumDOutMax=[]  DifferentiatorOutMin=[]  DifferentiatorOutMax=[]  FilterDiffOutCoefMin=[]  FilterDiffOutCoefMax=[]  ReciprocalOutMin=[]  ReciprocalOutMax=[]  SumDenOutMin=[]  SumDenOutMax=[]  SumNumOutMin=[]  SumNumOutMax=[]  DivideOutMin=[]  DivideOutMax=[]  UdiffTsProdOutMin=[]  UdiffTsProdOutMax=[]  NTsProdOutMin=[]  NTsProdOutMax=[]  UintegralTsProdOutMin=[]  UintegralTsProdOutMax=[]  UngainTsProdOutMin=[]  UngainTsProdOutMax=[]  ClampingZeroOutDataTypeStr=Inherit: Inherit via back propagation  ClampingZeroOutMin=[]  ClampingZeroOutMax=[]  FilterDenConstantOutDataTypeStr=Inherit: Inherit via back propagation  FilterDenConstantOutMin=[]  FilterDenConstantOutMax=[]  PCopyOutDataTypeStr=Inherit: Inherit via back propagation  PCopyOutMin=[]  PCopyOutMax=[]  NCopyOutDataTypeStr=Inherit: Inherit via back propagation  NCopyOutMin=[]  NCopyOutMax=[]  IntegratorContinuousStateAttributes=''  IntegratorStateMustResolveToSignalObject=off  IntegratorRTWStateStorageClass=Auto  FilterContinuousStateAttributes=''  FilterStateMustResolveToSignalObject=off  FilterRTWStateStorageClass=Auto  ParallelPVariant=InternalParameters  IdealPVariant=Disabled  IVariant=InternalParameters  DVariant=Disabled  IntegratorVariant=Continuous  SatVariant=Disabled  AWVariant=Passthrough  PCopyVariant=Disabled  TRVariant=Disabled  FdbkBlocksVariant=Forward  IdealPFdbkVariant=Disabled  SatFdbkVariant=Disabled  DerivativeFilterVariant=Disabled  NVariant=Disabled  NCopyVariant=Disabled_SignalSpec  FilterICVariant=Disabled  IntegratorICVariant=InternalICs  ExternalResetVariant=ExternalReset  TRSumVariant=Passthrough  SumFdbkVariant=Disabled  SumVariant=Sum_PI  TsampFilterVariant=InternalTs  TsampNgainVariant=Passthrough  TsampIntegralVariant=Disabled_SignalSpec  ExternalSaturationOutDataTypeStr=Inherit: Same as second input  DerivativeSourceVariant=Disabled  PreIntVariant=InternalPreInt
  dP : Outport
  tag scope: m4=global
  wires:
  Multiply/1 -> dP/1
  df/1 -> LTI System8/1
  PID Controller/1 -> Multiply/1
  [resetI] -> PID Controller/2
  LTI System8/1 -> [m4], PID Controller/1

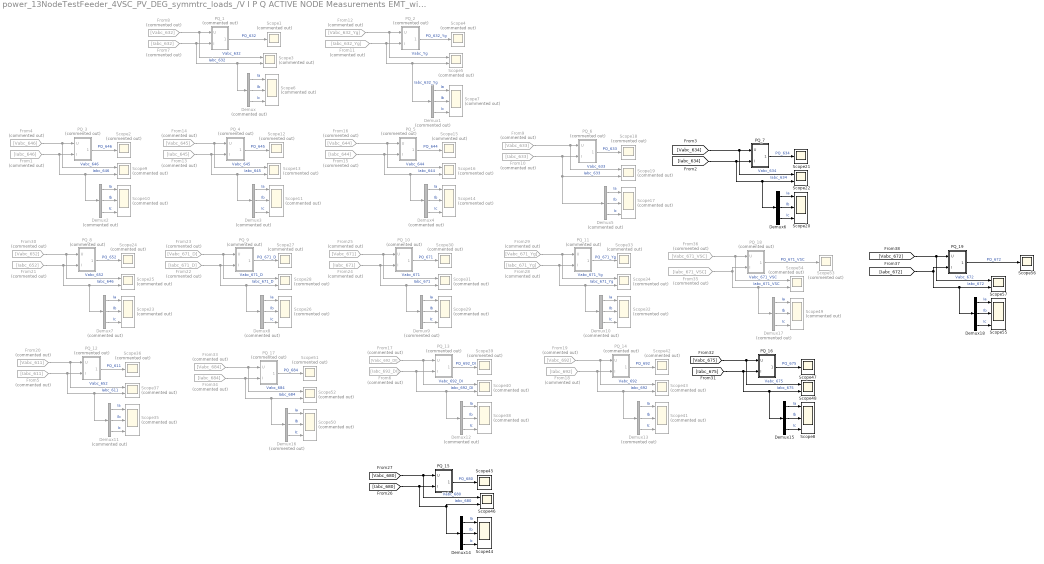
== system power_13NodeTestFeeder_4VSC_PV_DEG_symmtrc_loads_/V I P Q ACTIVE NODE Measurements EMT_with scopes_without_logsout1 ==
  Demux{,1..5,7..13,16..17} (15 alike) : Demux  Commented=on  Outputs=3
  Demux{6,14..15,18} (4 alike) : Demux  Outputs=3
  From1 : From  Commented=on  GotoTag=Iabc_646  TagVisibility=global
  From10 : From  Commented=on  GotoTag=Iabc_633  TagVisibility=global
  From11 : From  Commented=on  GotoTag=Iabc_632_Yg  TagVisibility=global
  From12 : From  Commented=on  GotoTag=Vabc_632_Yg  TagVisibility=global
  From13 : From  Commented=on  GotoTag=Iabc_645  TagVisibility=global
  From14 : From  Commented=on  GotoTag=Vabc_645  TagVisibility=global
  From15 : From  Commented=on  GotoTag=Iabc_644  TagVisibility=global
  From16 : From  Commented=on  GotoTag=Vabc_644  TagVisibility=global
  From17 : From  Commented=on  GotoTag=Vabc_692_DI  TagVisibility=global
  From18 : From  Commented=on  GotoTag=Iabc_692  TagVisibility=global
  From19 : From  Commented=on  GotoTag=Vabc_692  TagVisibility=global
  From20 : From  Commented=on  GotoTag=Vabc_611  TagVisibility=global
  From21 : From  Commented=on  GotoTag=Iabc_652  TagVisibility=global
  From22 : From  Commented=on  GotoTag=Iabc_671_D  TagVisibility=global
  From23 : From  Commented=on  GotoTag=Vabc_671_D  TagVisibility=global
  From24 : From  Commented=on  GotoTag=Iabc_671  TagVisibility=global
  From25 : From  Commented=on  GotoTag=Vabc_671  TagVisibility=global
  From28 : From  Commented=on  GotoTag=Iabc_671_Yg  TagVisibility=global
  From29 : From  Commented=on  GotoTag=Vabc_671_Yg  TagVisibility=global
  From30 : From  Commented=on  GotoTag=Vabc_652  TagVisibility=global
  From33 : From  Commented=on  GotoTag=Vabc_684  TagVisibility=global
  From34 : From  Commented=on  GotoTag=Iabc_684  TagVisibility=global
  From35 : From  Commented=on  GotoTag=Iabc_671_VSC  TagVisibility=global
  From36 : From  Commented=on  GotoTag=Vabc_671_VSC  TagVisibility=global
  From4 : From  Commented=on  GotoTag=Vabc_646  TagVisibility=global
  From5 : From  Commented=on  GotoTag=Iabc_611  TagVisibility=global
  From6 : From  Commented=on  GotoTag=Iabc_692_DI  TagVisibility=global
  From7 : From  Commented=on  GotoTag=Iabc_632  TagVisibility=global
  From8 : From  Commented=on  GotoTag=Vabc_632  TagVisibility=global
  From9 : From  Commented=on  GotoTag=Vabc_633  TagVisibility=global
  PQ_1 : Subsystem  Commented=on
  PQ_10 : Subsystem  Commented=on
  PQ_11 : Subsystem  Commented=on
  PQ_12 : Subsystem  Commented=on
  PQ_13 : Subsystem  Commented=on
  PQ_14 : Subsystem  Commented=on
  PQ_15 : Subsystem
  PQ_16 : Subsystem
  PQ_17 : Subsystem  Commented=on
  PQ_18 : Subsystem  Commented=on
  PQ_19 : Subsystem
  PQ_2 : Subsystem  Commented=on
  PQ_3 : Subsystem  Commented=on
  PQ_4 : Subsystem  Commented=on
  PQ_5 : Subsystem  Commented=on
  PQ_6 : Subsystem  Commented=on
  PQ_7 : Subsystem
  PQ_8 : Subsystem  Commented=on
  PQ_9 : Subsystem  Commented=on
  Scope{1..2,4,12,15,18,24,27,30,33,36,39,42,51,53} (15 alike) : Scope  Commented=on
  Scope{6..7,10..11,14,17,23,26,29,32,35,38,41,49..50} (15 alike) : Scope  Commented=on  NumInputPorts=3
  Scope{3,5,9,13,16,19,25,28,31,34,37,40,43,52,54} (15 alike) : Scope  Commented=on  NumInputPorts=2
  Scope{8,20,44,55} (4 alike) : Scope  NumInputPorts=3
  Scope{21,45,47,56} (4 alike) : Scope
  Scope{22,46,48,57} (4 alike) : Scope  NumInputPorts=2
  wires:
  From7/1 -> Demux/1, Scope3/2, PQ_1/2(I)  "Iabc_632"
  PQ_1/1(PQ) -> Scope1/1  "PQ_632"
  From8/1 -> Scope3/1, PQ_1/1(U)  "Vabc_632"
  PQ_2/1(PQ) -> Scope4/1  "PQ_632_Yg"
  From12/1 -> Scope5/1, PQ_2/1(U)  "Vabc_Yg"
  Demux/1 -> Scope6/1  "Ia"
  Demux/2 -> Scope6/2  "Ib"
  Demux/3 -> Scope6/3  "Ic"
  From11/1 -> Demux1/1, Scope5/2, PQ_2/2(I)  "Iabc_632_Yg"
  Demux1/1 -> Scope7/1  "Ia"
  Demux1/3 -> Scope7/3  "Ic"
  Demux1/2 -> Scope7/2  "Ib"
  Demux2/1 -> Scope10/1  "Ia"
  Demux2/2 -> Scope10/2  "Ib"
  From1/1 -> Scope9/2, Demux2/1, PQ_3/2(I)  "Iabc_646"
  PQ_3/1(PQ) -> Scope2/1  "PQ_646"
  From4/1 -> Scope9/1, PQ_3/1(U)  "Vabc_646"
  Demux2/3 -> Scope10/3  "Ic"
  Demux3/2 -> Scope11/2  "Ib"
  Demux3/1 -> Scope11/1  "Ia"
  Demux3/3 -> Scope11/3  "Ic"
  PQ_4/1(PQ) -> Scope12/1  "PQ_645"
  From14/1 -> Scope13/1, PQ_4/1(U)  "Vabc_645"
  From13/1 -> Scope13/2, Demux3/1, PQ_4/2(I)  "Iabc_645"
  Demux4/2 -> Scope14/2  "Ib"
  Demux4/1 -> Scope14/1  "Ia"
  Demux4/3 -> Scope14/3  "Ic"
  PQ_5/1(PQ) -> Scope15/1  "PQ_644"
  From16/1 -> Scope16/1, PQ_5/1(U)  "Vabc_644"
  From15/1 -> Scope16/2, Demux4/1, PQ_5/2(I)  "Iabc_644"
  Demux5/3 -> Scope17/3  "Ic"
  PQ_6/1(PQ) -> Scope18/1  "PQ_633"
  Demux5/1 -> Scope17/1  "Ia"
  Demux5/2 -> Scope17/2  "Ib"
  Demux6/2 -> Scope20/2  "Ib"
  PQ_7/1(PQ) -> Scope21/1  "PQ_634"
  Demux6/3 -> Scope20/3  "Ic"
  Demux6/1 -> Scope20/1  "Ia"
  [Iabc_634] -> Scope22/2, Demux6/1, PQ_7/2(I)  "Iabc_634"
  [Vabc_634] -> Scope22/1, PQ_7/1(U)  "Vabc_634"
  Demux7/2 -> Scope23/2  "Ib"
  Demux7/1 -> Scope23/1  "Ia"
  Demux7/3 -> Scope23/3  "Ic"
  PQ_8/1(PQ) -> Scope24/1  "PQ_652"
  From30/1 -> Scope25/1, PQ_8/1(U)  "Vabc_652"
  From21/1 -> Scope25/2, Demux7/1, PQ_8/2(I)  "Iabc_646"
  Demux8/2 -> Scope26/2  "Ib"
  Demux8/1 -> Scope26/1  "Ia"
  Demux8/3 -> Scope26/3  "Ic"
  PQ_9/1(PQ) -> Scope27/1  "PQ_671_D"
  From23/1 -> Scope28/1, PQ_9/1(U)  "Vabc_671_D"
  From22/1 -> Scope28/2, Demux8/1, PQ_9/2(I)  "Iabc_671_D"
  Demux9/2 -> Scope29/2  "Ib"
  Demux9/1 -> Scope29/1  "Ia"
  Demux9/3 -> Scope29/3  "Ic"
  PQ_10/1(PQ) -> Scope30/1  "PQ_671"
  From25/1 -> Scope31/1, PQ_10/1(U)  "Vabc_671"
  From24/1 -> Scope31/2, Demux9/1, PQ_10/2(I)  "Iabc_671"
  Demux10/2 -> Scope32/2  "Ib"
  Demux10/1 -> Scope32/1  "Ia"
  Demux10/3 -> Scope32/3  "Ic"
  PQ_11/1(PQ) -> Scope33/1  "PQ_671_Yg"
  From29/1 -> Scope34/1, PQ_11/1(U)  "Vabc_671_Yg"
  From28/1 -> Scope34/2, Demux10/1, PQ_11/2(I)  "Iabc_671_Yg"
  From20/1 -> Scope37/1, PQ_12/1(U)  "Vabc_652"
  PQ_12/1(PQ) -> Scope36/1  "PQ_611"
  Demux11/3 -> Scope35/3  "Ic"
  Demux11/1 -> Scope35/1  "Ia"
  From5/1 -> Scope37/2, Demux11/1, PQ_12/2(I)  "Iabc_611"
  Demux11/2 -> Scope35/2  "Ib"
  PQ_13/1(PQ) -> Scope39/1  "PQ_692_DI"
  Demux12/3 -> Scope38/3  "Ic"
  From17/1 -> Scope40/1, PQ_13/1(U)  "Vabc_692_DI"
  Demux12/2 -> Scope38/2  "Ib"
  Demux12/1 -> Scope38/1  "Ia"
  From6/1 -> PQ_13/2(I), Scope40/2, Demux12/1  "Iabc_692_DI"
  PQ_14/1(PQ) -> Scope42/1  "PQ_692"
  Demux13/3 -> Scope41/3  "Ic"
  From19/1 -> Scope43/1, PQ_14/1(U)  "Vabc_692"
  Demux13/2 -> Scope41/2  "Ib"
  Demux13/1 -> Scope41/1  "Ia"
  From18/1 -> Scope43/2, Demux13/1, PQ_14/2(I)  "Iabc_692"
  Demux14/1 -> Scope44/1  "Ia"
  [Vabc_680] -> Scope46/1, PQ_15/1(U)  "Vabc_680"
  [Iabc_680] -> Scope46/2, Demux14/1, PQ_15/2(I)  "Iabc_680"
  PQ_15/1(PQ) -> Scope45/1  "PQ_680"
  Demux14/2 -> Scope44/2  "Ib"
  Demux14/3 -> Scope44/3  "Ic"
  [Iabc_675] -> Scope48/2, Demux15/1, PQ_16/2(I)  "Iabc_675"
  Demux15/3 -> Scope8/3  "Ic"
  Demux15/1 -> Scope8/1  "Ia"
  Demux15/2 -> Scope8/2  "Ib"
  PQ_16/1(PQ) -> Scope47/1  "PQ_675"
  [Vabc_675] -> Scope48/1, PQ_16/1(U)  "Vabc_675"
  From10/1 -> Demux5/1, Scope19/2, PQ_6/2(I)  "Iabc_633"
  From9/1 -> Scope19/1, PQ_6/1(U)  "Vabc_633"
  From33/1 -> Scope52/1, PQ_17/1(U)  "Vabc_684"
  Demux16/1 -> Scope50/1  "Ia"
  Demux16/3 -> Scope50/3  "Ic"
  From34/1 -> Scope52/2, Demux16/1, PQ_17/2(I)  "Iabc_684"
  Demux16/2 -> Scope50/2  "Ib"
  PQ_17/1(PQ) -> Scope51/1  "PQ_684"
  Demux17/1 -> Scope49/1  "Ia"
  PQ_18/1(PQ) -> Scope53/1  "PQ_671_VSC"
  From36/1 -> Scope54/1, PQ_18/1(U)  "Vabc_671_VSC"
  Demux17/3 -> Scope49/3  "Ic"
  From35/1 -> PQ_18/2(I), Scope54/2, Demux17/1  "Iabc_671_VSC"
  Demux17/2 -> Scope49/2  "Ib"
  Demux18/1 -> Scope55/1  "Ia"
  Demux18/3 -> Scope55/3  "Ic"
  Demux18/2 -> Scope55/2  "Ib"
  [Iabc_672] -> PQ_19/2(I), Scope57/2, Demux18/1  "Iabc_672"
  [Vabc_672] -> Scope57/1, PQ_19/1(U)  "Vabc_672"
  PQ_19/1(PQ) -> Scope56/1  "PQ_672"

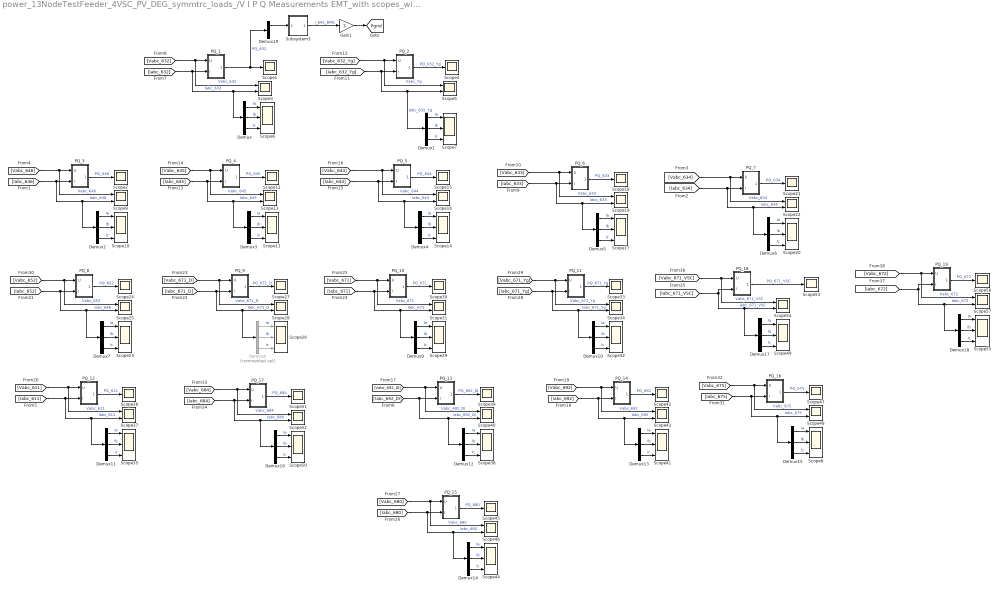
== system power_13NodeTestFeeder_4VSC_PV_DEG_symmtrc_loads_/V I P Q Measurements EMT_with scopes_without_logsout ==
  Demux{,1..7,9..18} (18 alike) : Demux  Outputs=3
  Demux19 : Demux  Outputs=2
  Demux8 : Demux  Commented=on  Outputs=3
  Gain1 : Gain  Gain=3
  PQ_1 : Subsystem
  PQ_10 : Subsystem
  PQ_11 : Subsystem
  PQ_12 : Subsystem
  PQ_13 : Subsystem
  PQ_14 : Subsystem
  PQ_15 : Subsystem
  PQ_16 : Subsystem
  PQ_17 : Subsystem
  PQ_18 : Subsystem
  PQ_19 : Subsystem
  PQ_2 : Subsystem
  PQ_3 : Subsystem
  PQ_4 : Subsystem
  PQ_5 : Subsystem
  PQ_6 : Subsystem
  PQ_7 : Subsystem
  PQ_8 : Subsystem
  PQ_9 : Subsystem
  Scope{1..2,4,12,15,18,21,24,27,30,33,36,39,42,45,47,51,53,56} (19 alike) : Scope
  Scope{6..8,10..11,14,17,20,23,26,29,32,35,38,41,44,49..50,55} (19 alike) : Scope  NumInputPorts=3
  Scope{3,5,9,13,16,19,22,25,28,31,34,37,40,43,46,48,52,54,57} (19 alike) : Scope  NumInputPorts=2
  Subsystem3 : Subsystem  mask{fg=fg, Vrms0=0}
      mask prompts: fg "Frequency"; Vrms0 "Initial value"
      mask Display: disp('RMS')
  tag scope: Pgrid=global
  wires:
  [Iabc_632] -> Demux/1, Scope3/2, PQ_1/2(I)  "Iabc_632"
  PQ_1/1(PQ) -> Demux19/1, Scope1/1  "PQ_632"
  [Vabc_632] -> Scope3/1, PQ_1/1(U)  "Vabc_632"
  PQ_2/1(PQ) -> Scope4/1  "PQ_632_Yg"
  [Vabc_632_Yg] -> Scope5/1, PQ_2/1(U)  "Vabc_Yg"
  Demux/1 -> Scope6/1  "Ia"
  Demux/2 -> Scope6/2  "Ib"
  Demux/3 -> Scope6/3  "Ic"
  [Iabc_632_Yg] -> Demux1/1, Scope5/2, PQ_2/2(I)  "Iabc_632_Yg"
  Demux1/1 -> Scope7/1  "Ia"
  Demux1/3 -> Scope7/3  "Ic"
  Demux1/2 -> Scope7/2  "Ib"
  Demux2/1 -> Scope10/1  "Ia"
  Demux2/2 -> Scope10/2  "Ib"
  [Iabc_646] -> Scope9/2, Demux2/1, PQ_3/2(I)  "Iabc_646"
  PQ_3/1(PQ) -> Scope2/1  "PQ_646"
  [Vabc_646] -> Scope9/1, PQ_3/1(U)  "Vabc_646"
  Demux2/3 -> Scope10/3  "Ic"
  Demux3/2 -> Scope11/2  "Ib"
  Demux3/1 -> Scope11/1  "Ia"
  Demux3/3 -> Scope11/3  "Ic"
  PQ_4/1(PQ) -> Scope12/1  "PQ_645"
  [Vabc_645] -> Scope13/1, PQ_4/1(U)  "Vabc_645"
  [Iabc_645] -> Scope13/2, Demux3/1, PQ_4/2(I)  "Iabc_645"
  Demux4/2 -> Scope14/2  "Ib"
  Demux4/1 -> Scope14/1  "Ia"
  Demux4/3 -> Scope14/3  "Ic"
  PQ_5/1(PQ) -> Scope15/1  "PQ_644"
  [Vabc_644] -> Scope16/1, PQ_5/1(U)  "Vabc_644"
  [Iabc_644] -> Scope16/2, Demux4/1, PQ_5/2(I)  "Iabc_644"
  Demux5/3 -> Scope17/3  "Ic"
  PQ_6/1(PQ) -> Scope18/1  "PQ_633"
  Demux5/1 -> Scope17/1  "Ia"
  [Vabc_633] -> Scope19/1, PQ_6/1(U)  "Vabc_633"
  Demux5/2 -> Scope17/2  "Ib"
  [Iabc_633] -> Scope19/2, Demux5/1, PQ_6/2(I)  "Iabc_633"
  Demux6/2 -> Scope20/2  "Ib"
  PQ_7/1(PQ) -> Scope21/1  "PQ_634"
  Demux6/3 -> Scope20/3  "Ic"
  Demux6/1 -> Scope20/1  "Ia"
  [Iabc_634] -> Scope22/2, Demux6/1, PQ_7/2(I)  "Iabc_634"
  [Vabc_634] -> Scope22/1, PQ_7/1(U)  "Vabc_634"
  Demux7/2 -> Scope23/2  "Ib"
  Demux7/1 -> Scope23/1  "Ia"
  Demux7/3 -> Scope23/3  "Ic"
  PQ_8/1(PQ) -> Scope24/1  "PQ_652"
  [Vabc_652] -> Scope25/1, PQ_8/1(U)  "Vabc_652"
  [Iabc_652] -> Scope25/2, Demux7/1, PQ_8/2(I)  "Iabc_646"
  Demux8/2 -> Scope26/2  "Ib"
  Demux8/1 -> Scope26/1  "Ia"
  Demux8/3 -> Scope26/3  "Ic"
  PQ_9/1(PQ) -> Scope27/1  "PQ_671_D"
  [Vabc_671_D] -> Scope28/1, PQ_9/1(U)  "Vabc_671_D"
  [Iabc_671_D] -> Scope28/2, Demux8/1, PQ_9/2(I)  "Iabc_671_D"
  Demux9/2 -> Scope29/2  "Ib"
  Demux9/1 -> Scope29/1  "Ia"
  Demux9/3 -> Scope29/3  "Ic"
  PQ_10/1(PQ) -> Scope30/1  "PQ_671"
  [Vabc_671] -> Scope31/1, PQ_10/1(U)  "Vabc_671"
  [Iabc_671] -> Scope31/2, Demux9/1, PQ_10/2(I)  "Iabc_671"
  Demux10/2 -> Scope32/2  "Ib"
  Demux10/1 -> Scope32/1  "Ia"
  Demux10/3 -> Scope32/3  "Ic"
  PQ_11/1(PQ) -> Scope33/1  "PQ_671_Yg"
  [Vabc_671_Yg] -> Scope34/1, PQ_11/1(U)  "Vabc_671_Yg"
  [Iabc_671_Yg] -> Scope34/2, Demux10/1, PQ_11/2(I)  "Iabc_671_Yg"
  [Vabc_611] -> Scope37/1, PQ_12/1(U)  "Vabc_611"
  PQ_12/1(PQ) -> Scope36/1  "PQ_611"
  Demux11/3 -> Scope35/3  "Ic"
  Demux11/1 -> Scope35/1  "Ia"
  [Iabc_611] -> Scope37/2, Demux11/1, PQ_12/2(I)  "Iabc_611"
  Demux11/2 -> Scope35/2  "Ib"
  PQ_13/1(PQ) -> Scope39/1  "PQ_692_DI"
  Demux12/3 -> Scope38/3  "Ic"
  [Vabc_692_DI] -> Scope40/1, PQ_13/1(U)  "Vabc_692_DI"
  Demux12/2 -> Scope38/2  "Ib"
  Demux12/1 -> Scope38/1  "Ia"
  [Iabc_692_DI] -> PQ_13/2(I), Scope40/2, Demux12/1  "Iabc_692_DI"
  PQ_14/1(PQ) -> Scope42/1  "PQ_692"
  Demux13/3 -> Scope41/3  "Ic"
  [Vabc_692] -> Scope43/1, PQ_14/1(U)  "Vabc_692"
  Demux13/2 -> Scope41/2  "Ib"
  Demux13/1 -> Scope41/1  "Ia"
  [Iabc_692] -> Scope43/2, Demux13/1, PQ_14/2(I)  "Iabc_692"
  Demux14/1 -> Scope44/1  "Ia"
  [Vabc_680] -> Scope46/1, PQ_15/1(U)  "Vabc_680"
  [Iabc_680] -> Scope46/2, Demux14/1, PQ_15/2(I)  "Iabc_680"
  PQ_15/1(PQ) -> Scope45/1  "PQ_680"
  Demux14/2 -> Scope44/2  "Ib"
  Demux14/3 -> Scope44/3  "Ic"
  [Vabc_675] -> Scope48/1, PQ_16/1(U)  "Vabc_675"
  Demux15/3 -> Scope8/3  "Ic"
  PQ_16/1(PQ) -> Scope47/1  "PQ_675"
  Demux15/1 -> Scope8/1  "Ia"
  [Iabc_675] -> Scope48/2, Demux15/1, PQ_16/2(I)  "Iabc_675"
  Demux15/2 -> Scope8/2  "Ib"
  PQ_17/1(PQ) -> Scope51/1  "PQ_684"
  [Iabc_684] -> Scope52/2, Demux16/1, PQ_17/2(I)  "Iabc_684"
  Demux16/2 -> Scope50/2  "Ib"
  Demux16/3 -> Scope50/3  "Ic"
  Demux16/1 -> Scope50/1  "Ia"
  [Vabc_684] -> Scope52/1, PQ_17/1(U)  "Vabc_684"
  [Iabc_671_VSC] -> PQ_18/2(I), Scope54/2, Demux17/1  "Iabc_671_VSC"
  [Vabc_671_VSC] -> Scope54/1, PQ_18/1(U)  "Vabc_671_VSC"
  Demux17/3 -> Scope49/3  "Ic"
  PQ_18/1(PQ) -> Scope53/1  "PQ_671_VSC"
  Demux17/2 -> Scope49/2  "Ib"
  Demux17/1 -> Scope49/1  "Ia"
  Demux18/3 -> Scope55/3  "Ic"
  Demux18/1 -> Scope55/1  "Ia"
  [Vabc_672] -> Scope57/1, PQ_19/1(U)  "Vabc_672"
  PQ_19/1(PQ) -> Scope56/1  "PQ_672"
  [Iabc_672] -> PQ_19/2(I), Scope57/2, Demux18/1  "Iabc_672"
  Demux18/2 -> Scope55/2  "Ib"
  Demux19/1 -> Subsystem3/1(In1)
  Subsystem3/1(Out1) -> Gain1/1  "I_645_RMS"
  Gain1/1 -> [Pgrid]
